simulink model "LAB_02_26_SEPT_NORM"  (R2022b)
settings: Solver=VariableStepAuto  StartTime=0.0  StopTime=10.0  RelTol=1e-3
settings Model: Creator=maria  LastModifiedBy=maria

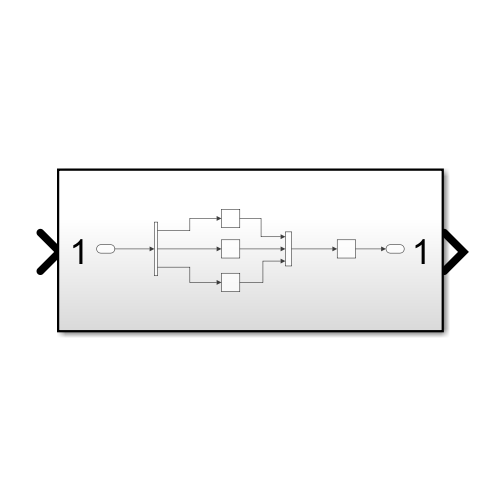
[thumbnail: Simulink's stored preview of the top-level diagram]
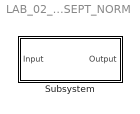
== system LAB_02_26_SEPT_NORM ==
  Subsystem : Subsystem

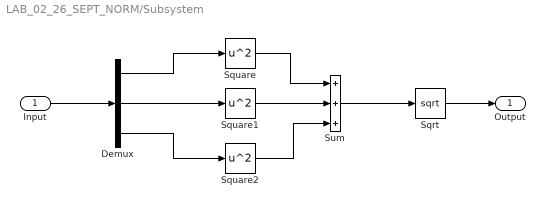
== system LAB_02_26_SEPT_NORM/Subsystem ==
  Input : Inport
  Demux : Demux  Outputs=3
  Sqrt : Sqrt
  Square : Math  Operator=square
  Square1 : Math  Operator=square
  Square2 : Math  Operator=square
  Sum : Sum  Inputs=+++
  Output : Outport
  wires:
  Square1/1 -> Sum/2
  Square/1 -> Sum/1
  Demux/3 -> Square2/1
  Input/1 -> Demux/1
  Sum/1 -> Sqrt/1
  Demux/1 -> Square/1
  Sqrt/1 -> Output/1
  Square2/1 -> Sum/3
  Demux/2 -> Square1/1
